simulink model "NDM200_Spindel_Kue_V1"  (Simulink 7.6)
settings: Solver=ode45  StartTime=0.0  StopTime=SimulTime  RelTol=1e-3
values from neighbouring files (symbols this model uses):
  n1 = 380/0.78    (= 487.179487179)    [ParametersGM.m]
  n2 = 1100/0.7    (= 1571.42857143)    [ParametersGM.m]
  p = 500/0.8    (= 625)    [ParametersGM.m]
  sb = 5.67*(10^-8)    (= 5.67e-08)    [ParametersGM.m]
  T_amb = 296    [ParametersGM.m]
  Venti_n2 = 273+40    (= 313)    [ParametersGM.m]
undefined symbols (not defined in the file or in its folder): Job, magnitude, MainDrive, MainDriveCooling
libraries: simulink x1
settings Model: Creator=conid  LastModifiedBy=conid

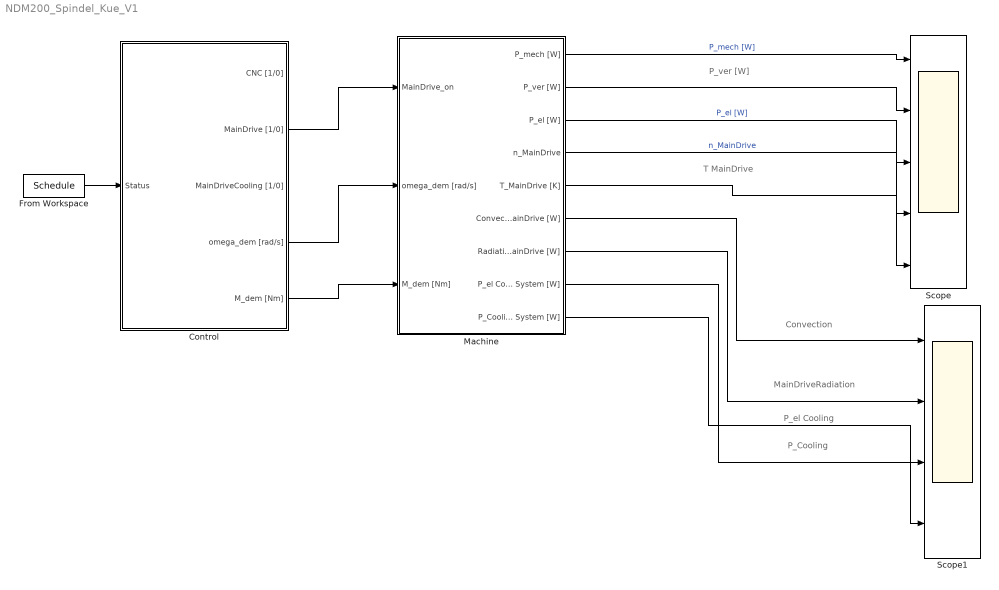
== system NDM200_Spindel_Kue_V1 ==
  note: P_ver [W]
  note: MainDriveRadiation
  note: Convection
  note: T MainDrive
  note: P_el Cooling
  note: P_Cooling
  Control : Subsystem  TreatAsAtomicUnit=on  mask{CNC=[0 1 1 1 1], MainDrive=[0 1 1 1 1], MainDriveCooling=[0 1 1 1 1], Job=Job}
      mask prompts: CNC "Cabinet"; MainDrive "Main Drive"; MainDriveCooling "Main Drive Cooling"; Job "Job Struct"
      mask help:
      | Controls the components of the machine:
      |
      | Status:
      |     0. Off
      |     1. Standby
      |     2. Warmup
      |     3. Setting
      |     4. Machining
      |
      | If the status is machining, the job defined as
      |     - Job.time
      |     - Job.omega_dem
      |     - Job.M_dem
      | will be runned, and repeated.
      mask TabNameString: Status,Status,Status,Job
  From Workspace : FromWorkspace  VariableName=Schedule  SampleTime=0  Interpolate=off  OutputAfterFinalValue=Holding final value
  Machine : Subsystem  TreatAsAtomicUnit=on
  Scope : Scope  NumInputPorts=5
      settings: TickLabels=on  YMin=-5~-5~-5~-5~-5  YMax=5~5~5~5~5  SaveName=Scp_MainDrive
  Scope1 : Scope  NumInputPorts=4
      settings: TickLabels=on  YMin=-5~-5~-5~-5  YMax=5~5~5~5  SaveName=Scp_MainDrive1
  wires:
  Machine/1(P_mech [W]) -> Scope/1  "P_mech [W]"
  Machine/2(P_ver [W]) -> Scope/2
  Machine/3(P_el [W]) -> Scope/3  "P_el [W]"
  Machine/4(n_MainDrive) -> Scope/4  "n_MainDrive"
  From Workspace/1 -> Control/1(Status)
  Control/5(M_dem [Nm]) -> Machine/3(M_dem [Nm])
  Control/4(omega_dem [rad/s]) -> Machine/2(omega_dem [rad/s])
  Control/2(MainDrive [1/0]) -> Machine/1(MainDrive_on)
  Machine/5(T_MainDrive [K]) -> Scope/5
  Machine/6(ConvectionMainDrive [W]) -> Scope1/1
  Machine/7(RadiationMainDrive [W]) -> Scope1/2
  Machine/8(P_el Cooling System [W]) -> Scope1/3
  Machine/9(P_Cooling System [W]) -> Scope1/4

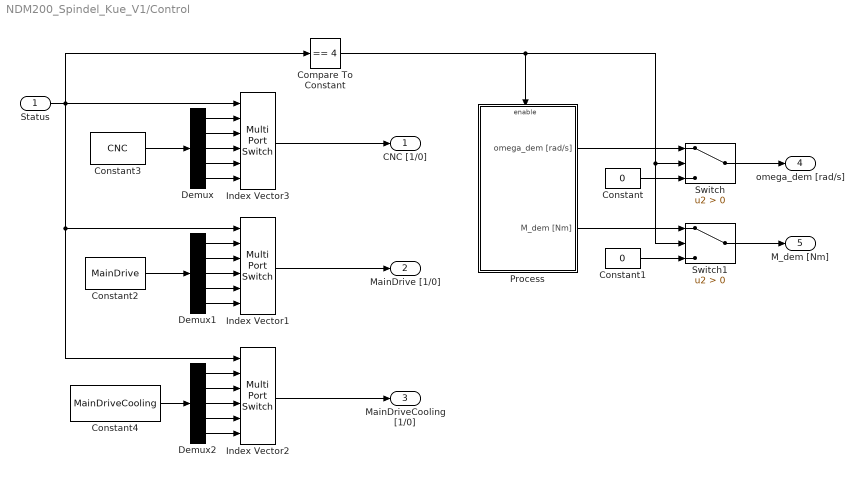
== system NDM200_Spindel_Kue_V1/Control ==
  Status : Inport
  Compare To Constant : simulink/Logic and Bit Operations/Compare To Constant  SystemSampleTime=-1  relop===  const=4  LogicOutDataTypeMode=uint8
  Constant : Constant  Value=0
  Constant1 : Constant  Value=0
  Constant2 : Constant  Value=MainDrive
  Constant3 : Constant  Value=CNC
  Constant4 : Constant  Value=MainDriveCooling
  Demux : Demux  Outputs=5
  Demux1 : Demux  Outputs=5
  Demux2 : Demux  Outputs=5
  Index Vector1 : MultiPortSwitch  DataPortOrder=Zero-based contiguous  Inputs=5  zeroidx=on
  Index Vector2 : MultiPortSwitch  DataPortOrder=Zero-based contiguous  Inputs=5  zeroidx=on
  Index Vector3 : MultiPortSwitch  DataPortOrder=Zero-based contiguous  Inputs=5  zeroidx=on
  Process : Subsystem  TreatAsAtomicUnit=on
  Switch : Switch  Criteria=u2 > Threshold
  Switch1 : Switch  Criteria=u2 > Threshold
  CNC [1/0] : Outport
  MainDrive [1/0] : Outport  Port=2
  MainDriveCooling [1/0] : Outport  Port=3
  omega_dem [rad/s] : Outport  Port=4
  M_dem [Nm] : Outport  Port=5
  wires:
  Status/1 -> Index Vector3/1, Index Vector2/1, Index Vector1/1, Compare To Constant/1
  Demux/1 -> Index Vector3/2
  Demux/2 -> Index Vector3/3
  Demux/3 -> Index Vector3/4
  Demux/4 -> Index Vector3/5
  Demux/5 -> Index Vector3/6
  Index Vector3/1 -> CNC [1/0]/1
  Demux1/1 -> Index Vector1/2
  Demux1/2 -> Index Vector1/3
  Demux1/3 -> Index Vector1/4
  Demux1/4 -> Index Vector1/5
  Demux1/5 -> Index Vector1/6
  Index Vector1/1 -> MainDrive [1/0]/1
  Demux2/1 -> Index Vector2/2
  Demux2/2 -> Index Vector2/3
  Demux2/3 -> Index Vector2/4
  Demux2/4 -> Index Vector2/5
  Demux2/5 -> Index Vector2/6
  Index Vector2/1 -> MainDriveCooling [1/0]/1
  Compare To Constant/1 -> Process/Enable, Switch1/2, Switch/2
  Process/1(omega_dem [rad/s]) -> Switch/1
  Constant/1 -> Switch/3
  Process/2(M_dem [Nm]) -> Switch1/1
  Constant1/1 -> Switch1/3
  Switch/1 -> omega_dem [rad/s]/1
  Switch1/1 -> M_dem [Nm]/1
  Constant3/1 -> Demux/1
  Constant2/1 -> Demux1/1
  Constant4/1 -> Demux2/1

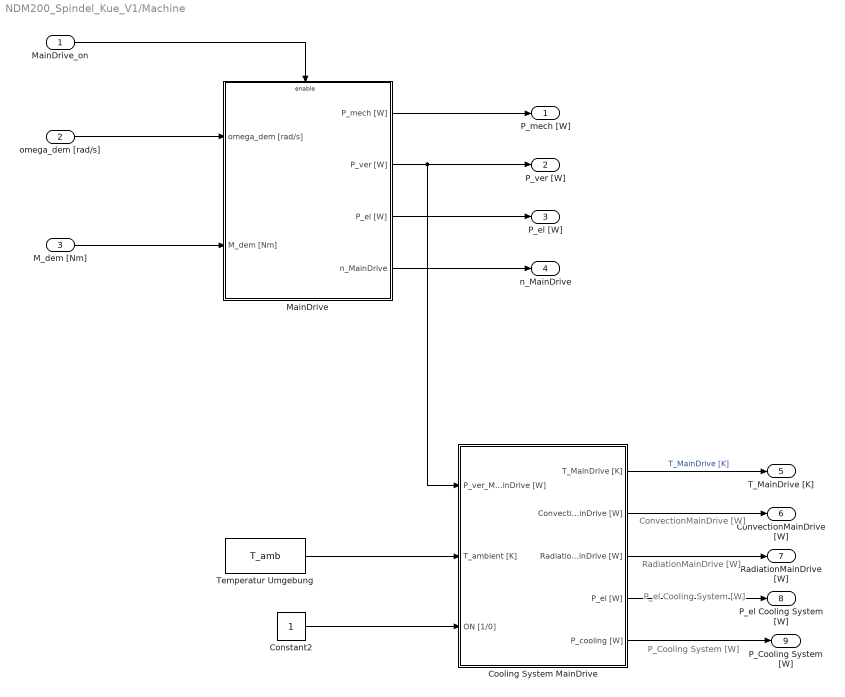
== system NDM200_Spindel_Kue_V1/Machine ==
  note: ConvectionMainDrive [W]
  note: RadiationMainDrive [W]
  note: P_el Cooling System [W]
  note: P_Cooling System [W]
  MainDrive_on : Inport
  omega_dem [rad/s] : Inport  Port=2
  M_dem [Nm] : Inport  Port=3
  Constant2 : Constant
  Cooling System MainDrive : Subsystem  TreatAsAtomicUnit=on
  MainDrive : Subsystem  TreatAsAtomicUnit=on
  Temperatur Umgebung : Constant  Value=T_amb
  P_mech [W] : Outport
  P_ver [W] : Outport  Port=2
  P_el [W] : Outport  Port=3
  n_MainDrive : Outport  Port=4
  T_MainDrive [K] : Outport  Port=5
  ConvectionMainDrive [W] : Outport  Port=6
  RadiationMainDrive [W] : Outport  Port=7
  P_el Cooling System [W] : Outport  Port=8
  P_Cooling System [W] : Outport  Port=9
  wires:
  MainDrive/2(P_ver [W]) -> P_ver [W]/1, Cooling System MainDrive/1(P_ver_MainDrive [W])
  MainDrive/1(P_mech [W]) -> P_mech [W]/1
  MainDrive/3(P_el [W]) -> P_el [W]/1
  MainDrive/4(n_MainDrive) -> n_MainDrive/1
  MainDrive_on/1 -> MainDrive/Enable
  M_dem [Nm]/1 -> MainDrive/2(M_dem [Nm])
  omega_dem [rad/s]/1 -> MainDrive/1(omega_dem [rad/s])
  Temperatur Umgebung/1 -> Cooling System MainDrive/2(T_ambient [K])
  Cooling System MainDrive/1(T_MainDrive [K]) -> T_MainDrive [K]/1  "T_MainDrive [K]"
  Cooling System MainDrive/2(ConvectionMainDrive [W]) -> ConvectionMainDrive [W]/1
  Cooling System MainDrive/3(RadiationMainDrive [W]) -> RadiationMainDrive [W]/1
  Cooling System MainDrive/4(P_el [W]) -> P_el Cooling System [W]/1
  Cooling System MainDrive/5(P_cooling [W]) -> P_Cooling System [W]/1
  Constant2/1 -> Cooling System MainDrive/3(ON [1/0])

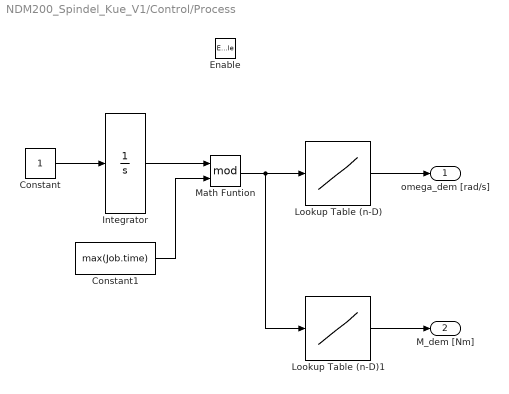
== system NDM200_Spindel_Kue_V1/Control/Process ==
  Enable : EnablePort
  Constant : Constant
  Constant1 : Constant  Value=max(Job.time)
  Integrator : Integrator
  Lookup Table (n-D) : Lookup_n-D  NumberOfTableDimensions=1  BreakpointsForDimension1=Job.time  Table=Job.omega_dem  InterpMethod=None - Flat  ExtrapMethod=Cubic spline  InputSameDT=on
  Lookup Table (n-D)1 : Lookup_n-D  NumberOfTableDimensions=1  BreakpointsForDimension1=Job.time  Table=Job.M_dem  InterpMethod=None - Flat  InputSameDT=on
  Math Funtion : Math  Operator=mod  SaturateOnIntegerOverflow=on
  omega_dem [rad/s] : Outport
  M_dem [Nm] : Outport  Port=2
  wires:
  Constant/1 -> Integrator/1
  Integrator/1 -> Math Funtion/1
  Math Funtion/1 -> Lookup Table (n-D)/1, Lookup Table (n-D)1/1
  Lookup Table (n-D)/1 -> omega_dem [rad/s]/1
  Lookup Table (n-D)1/1 -> M_dem [Nm]/1
  Constant1/1 -> Math Funtion/2

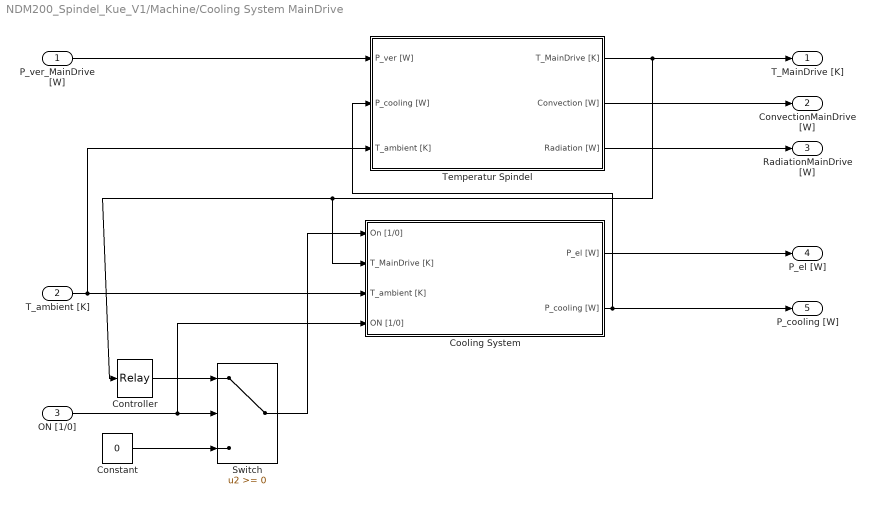
== system NDM200_Spindel_Kue_V1/Machine/Cooling System MainDrive ==
  P_ver_MainDrive [W] : Inport
  T_ambient [K] : Inport  Port=2
  ON [1/0] : Inport  Port=3
  Constant : Constant  Value=0
  Controller : Relay  OnSwitchValue=MainDriveCooling.Tmax  OffSwitchValue=MainDriveCooling.Tmin
  Cooling System : Subsystem
  Switch : Switch
  Temperatur Spindel : Subsystem
  T_MainDrive [K] : Outport
  ConvectionMainDrive [W] : Outport  Port=2
  RadiationMainDrive [W] : Outport  Port=3
  P_el [W] : Outport  Port=4
  P_cooling [W] : Outport  Port=5
  wires:
  P_ver_MainDrive [W]/1 -> Temperatur Spindel/1(P_ver [W])
  Constant/1 -> Switch/3
  ON [1/0]/1 -> Switch/2, Cooling System/4(ON [1/0])
  Controller/1 -> Switch/1
  Temperatur Spindel/1(T_MainDrive [K]) -> Controller/1, Cooling System/2(T_MainDrive [K]), T_MainDrive [K]/1
  Switch/1 -> Cooling System/1(On [1/0])
  T_ambient [K]/1 -> Cooling System/3(T_ambient [K]), Temperatur Spindel/3(T_ambient [K])
  Cooling System/2(P_cooling [W]) -> Temperatur Spindel/2(P_cooling [W]), P_cooling [W]/1
  Temperatur Spindel/2(Convection [W]) -> ConvectionMainDrive [W]/1
  Temperatur Spindel/3(Radiation [W]) -> RadiationMainDrive [W]/1
  Cooling System/1(P_el [W]) -> P_el [W]/1

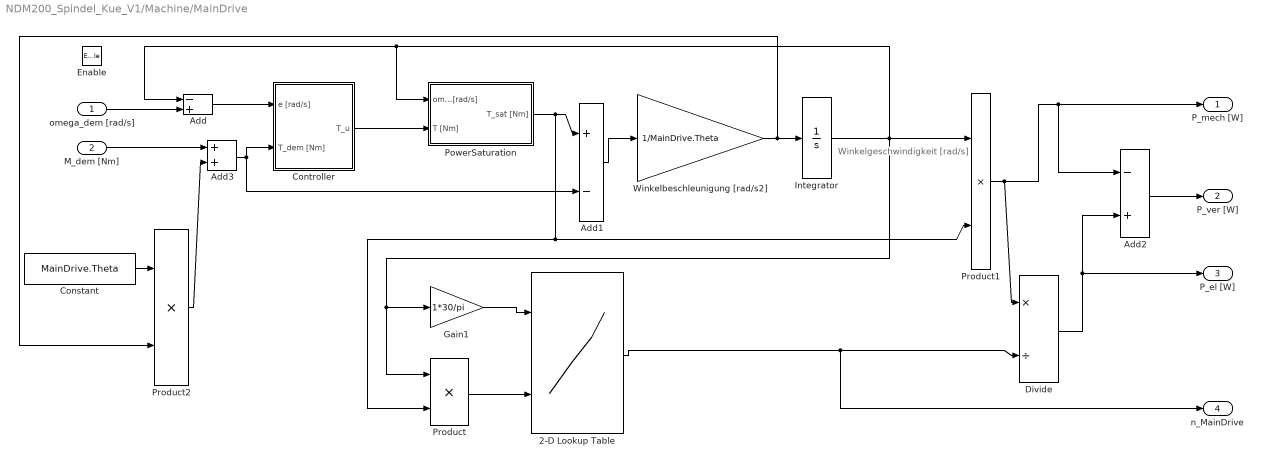
== system NDM200_Spindel_Kue_V1/Machine/MainDrive ==
  note: Winkelgeschwindigkeit [rad/s]
  omega_dem [rad/s] : Inport
  M_dem [Nm] : Inport  Port=2
  Enable : EnablePort
  2-D Lookup Table : Lookup_n-D  BreakpointsForDimension1=MainDrive.Tabelomega  BreakpointsForDimension2=MainDrive.TabelM  Table=MainDrive.Tabeleta  InterpMethod=Cubic spline  ExtrapMethod=Cubic spline  RndMeth=Simplest  InputSameDT=on
  Add : Sum  Inputs=-+
  Add1 : Sum  Inputs=+-
  Add2 : Sum  Inputs=-+
  Add3 : Sum
  Constant : Constant  Value=MainDrive.Theta
  Controller : Subsystem  TreatAsAtomicUnit=on
  Divide : Product  Inputs=*/
  Gain1 : Gain  Gain=1*30/pi
  Integrator : Integrator
  PowerSaturation : Subsystem  TreatAsAtomicUnit=on
  Product : Product  RndMeth=Zero
  Product1 : Product  RndMeth=Zero
  Product2 : Product  RndMeth=Zero
  Winkelbeschleunigung [rad/s2] : Gain  Gain=1/MainDrive.Theta
  P_mech [W] : Outport
  P_ver [W] : Outport  Port=2
  P_el [W] : Outport  Port=3
  n_MainDrive : Outport  Port=4
  wires:
  omega_dem [rad/s]/1 -> Add/2
  Add/1 -> Controller/1(e [rad/s])
  Controller/1(T_u) -> PowerSaturation/2(T [Nm])
  PowerSaturation/1(T_sat [Nm]) -> Add1/1, Product1/2, Product/2
  Add1/1 -> Winkelbeschleunigung [rad/s2]/1
  Winkelbeschleunigung [rad/s2]/1 -> Integrator/1, Product2/2
  Integrator/1 -> Product1/1, Add/1, PowerSaturation/1(omega [rad/s]), Product/1, Gain1/1
  Product1/1 -> Divide/1, P_mech [W]/1, Add2/1
  Add2/1 -> P_ver [W]/1
  Divide/1 -> Add2/2, P_el [W]/1
  2-D Lookup Table/1 -> Divide/2, n_MainDrive/1
  Product/1 -> 2-D Lookup Table/2
  Gain1/1 -> 2-D Lookup Table/1
  Constant/1 -> Product2/1
  Add3/1 -> Controller/2(T_dem [Nm]), Add1/2
  M_dem [Nm]/1 -> Add3/1
  Product2/1 -> Add3/2

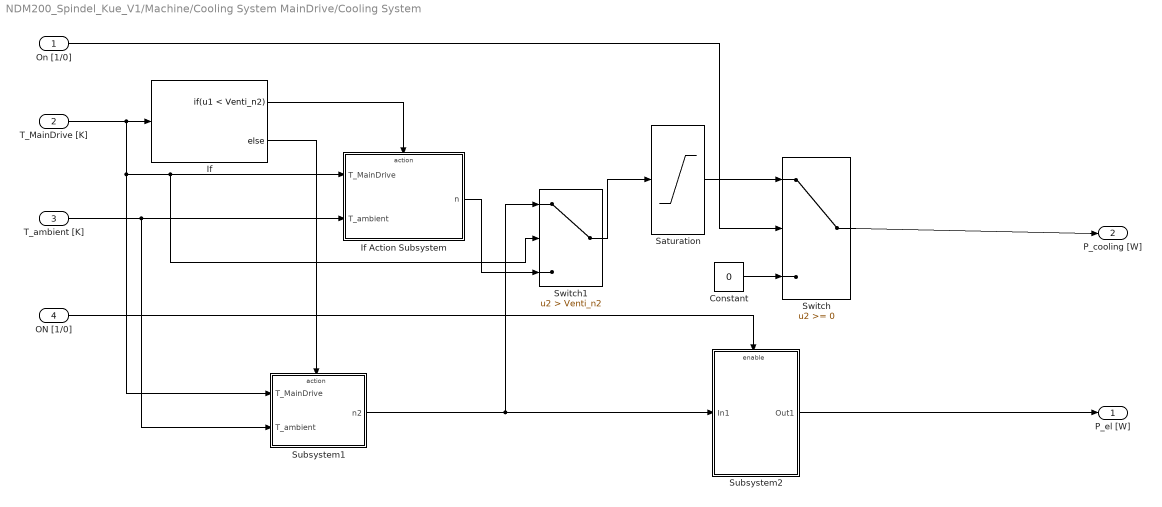
== system NDM200_Spindel_Kue_V1/Machine/Cooling System MainDrive/Cooling System ==
  On [1/0] : Inport
  T_MainDrive [K] : Inport  Port=2
  T_ambient [K] : Inport  Port=3
  ON [1/0] : Inport  Port=4
  Constant : Constant  Value=0
  If : If  IfExpression=u1 < Venti_n2
  If Action Subsystem : Subsystem  TreatAsAtomicUnit=on
  Saturation : Saturate  UpperLimit=12000  LowerLimit=0
  Subsystem1 : Subsystem
  Subsystem2 : Subsystem
  Switch : Switch
  Switch1 : Switch  Criteria=u2 > Threshold  Threshold=Venti_n2
  P_el [W] : Outport
  P_cooling [W] : Outport  Port=2
  wires:
  T_ambient [K]/1 -> Subsystem1/2(T_ambient), If Action Subsystem/2(T_ambient)
  Constant/1 -> Switch/3
  On [1/0]/1 -> Switch/2
  Saturation/1 -> Switch/1
  Switch/1 -> P_cooling [W]/1
  Subsystem2/1(Out1) -> P_el [W]/1
  T_MainDrive [K]/1 -> Subsystem1/1(T_MainDrive), If Action Subsystem/1(T_MainDrive), Switch1/2, If/1
  Subsystem1/1(n2) -> Subsystem2/1(In1), Switch1/1
  ON [1/0]/1 -> Subsystem2/Enable
  Switch1/1 -> Saturation/1
  If/1 -> If Action Subsystem/Action
  If/2 -> Subsystem1/Action
  If Action Subsystem/1(n) -> Switch1/3

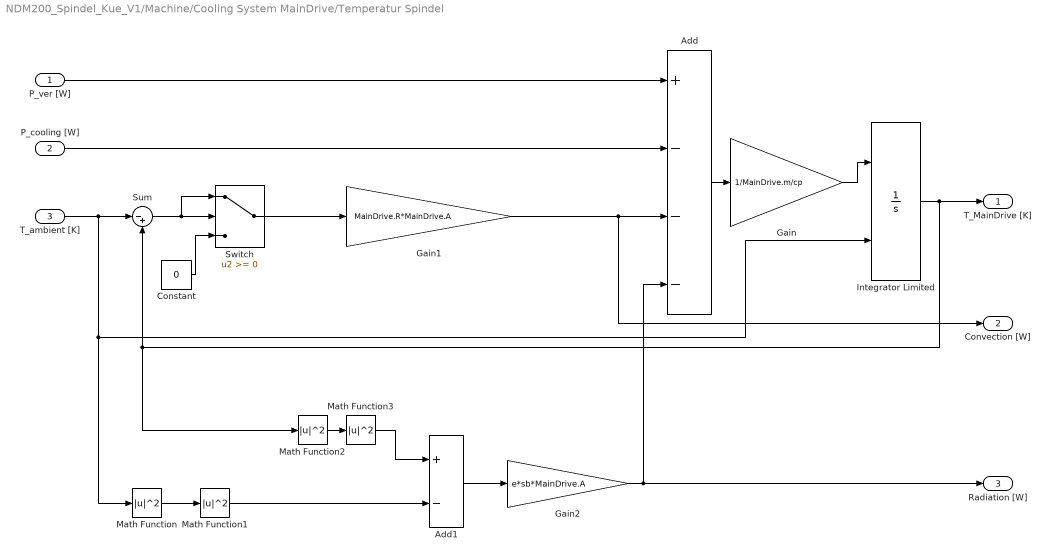
== system NDM200_Spindel_Kue_V1/Machine/Cooling System MainDrive/Temperatur Spindel ==
  P_ver [W] : Inport
  P_cooling [W] : Inport  Port=2
  T_ambient [K] : Inport  Port=3
  Add : Sum  Inputs=+---
  Add1 : Sum  Inputs=+-
  Constant : Constant  Value=0
  Gain : Gain  Gain=1/MainDrive.m/cp
  Gain1 : Gain  Gain=MainDrive.R*MainDrive.A
  Gain2 : Gain  Gain=e*sb*MainDrive.A
  Integrator Limited : Integrator  InitialConditionSource=external  LimitOutput=on
  Math Function{,1..3} (4 alike) : Math  Operator=magnitude^2  SaturateOnIntegerOverflow=on
  Sum : Sum  Inputs=|-+
  Switch : Switch
  T_MainDrive [K] : Outport
  Convection [W] : Outport  Port=2
  Radiation [W] : Outport  Port=3
  wires:
  P_ver [W]/1 -> Add/1
  Gain/1 -> Integrator Limited/1
  Gain1/1 -> Convection [W]/1, Add/3
  Integrator Limited/1 -> T_MainDrive [K]/1, Sum/2, Math Function2/1
  Add/1 -> Gain/1
  Math Function/1 -> Math Function1/1
  Gain2/1 -> Radiation [W]/1, Add/4
  P_cooling [W]/1 -> Add/2
  T_ambient [K]/1 -> Sum/1, Integrator Limited/2, Math Function/1
  Sum/1 -> Switch/2, Switch/1
  Constant/1 -> Switch/3
  Math Function2/1 -> Math Function3/1
  Add1/1 -> Gain2/1
  Math Function3/1 -> Add1/1
  Math Function1/1 -> Add1/2
  Switch/1 -> Gain1/1

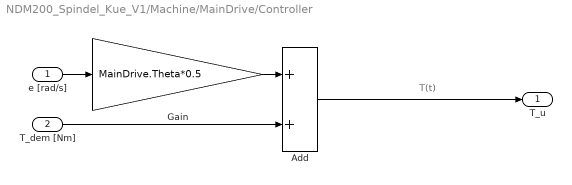
== system NDM200_Spindel_Kue_V1/Machine/MainDrive/Controller ==
  note: T(t)
  e [rad/s] : Inport
  T_dem [Nm] : Inport  Port=2
  Add : Sum
  Gain : Gain  Gain=MainDrive.Theta*0.5
  T_u : Outport
  wires:
  Add/1 -> T_u/1
  T_dem [Nm]/1 -> Add/2
  Gain/1 -> Add/1
  e [rad/s]/1 -> Gain/1

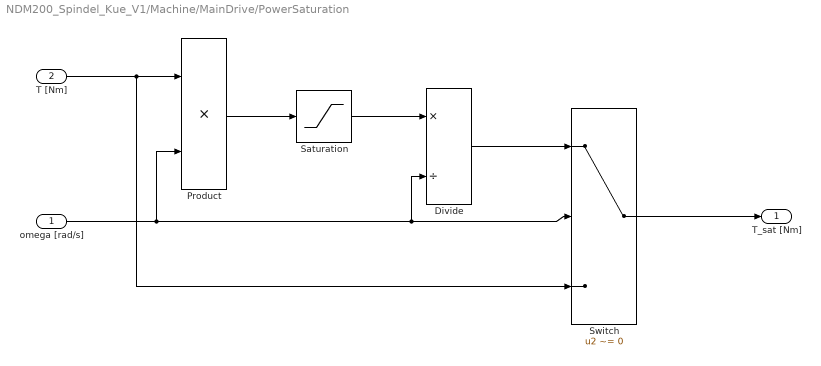
== system NDM200_Spindel_Kue_V1/Machine/MainDrive/PowerSaturation ==
  omega [rad/s] : Inport
  T [Nm] : Inport  Port=2
  Divide : Product  Inputs=*/
  Product : Product  RndMeth=Zero
  Saturation : Saturate  UpperLimit=MainDrive.Pmax  LowerLimit=-MainDrive.Pmax
  Switch : Switch  Criteria=u2 ~= 0
  T_sat [Nm] : Outport
  wires:
  Product/1 -> Saturation/1
  Saturation/1 -> Divide/1
  Divide/1 -> Switch/1
  Switch/1 -> T_sat [Nm]/1
  T [Nm]/1 -> Product/1, Switch/3
  omega [rad/s]/1 -> Switch/2, Divide/2, Product/2

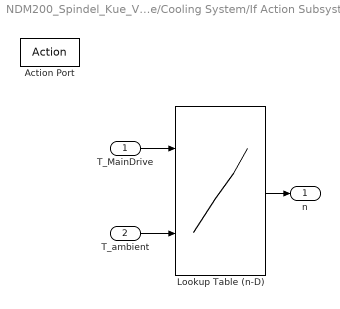
== system NDM200_Spindel_Kue_V1/Machine/Cooling System MainDrive/Cooling System/If Action Subsystem ==
  T_MainDrive : Inport
  T_ambient : Inport  Port=2
  Action Port : ActionPort  ActionType=then
  Lookup Table (n-D) : Lookup_n-D  BreakpointsForDimension1=MainDriveCooling.Air.T_int  BreakpointsForDimension2=MainDriveCooling.Air.T_ext  Table=MainDriveCooling.Air.P  InterpMethod=Cubic spline  ExtrapMethod=None - Clip  InputSameDT=on
  n : Outport
  wires:
  T_ambient/1 -> Lookup Table (n-D)/2
  T_MainDrive/1 -> Lookup Table (n-D)/1
  Lookup Table (n-D)/1 -> n/1

== system NDM200_Spindel_Kue_V1/Machine/Cooling System MainDrive/Cooling System/Subsystem1 ==
  T_MainDrive : Inport
  T_ambient : Inport  Port=2
  Action Port : ActionPort  ActionType=else
  Lookup Table (n-D)1 : Lookup_n-D  BreakpointsForDimension1=MainDriveCooling.Air.T_int  BreakpointsForDimension2=MainDriveCooling.Air.T_ext  Table=MainDriveCooling.Air.P_n2  InterpMethod=Cubic spline  ExtrapMethod=None - Clip  InputSameDT=on
  n2 : Outport
  wires:
  T_ambient/1 -> Lookup Table (n-D)1/2
  T_MainDrive/1 -> Lookup Table (n-D)1/1
  Lookup Table (n-D)1/1 -> n2/1

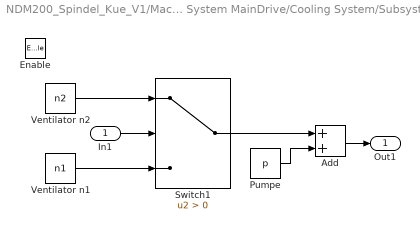
== system NDM200_Spindel_Kue_V1/Machine/Cooling System MainDrive/Cooling System/Subsystem2 ==
  In1 : Inport
  Enable : EnablePort
  Add : Sum
  Pumpe : Constant  Value=p
  Switch1 : Switch  Criteria=u2 > Threshold
  Ventilator n1 : Constant  Value=n1
  Ventilator n2 : Constant  Value=n2
  Out1 : Outport
  wires:
  Switch1/1 -> Add/1
  Ventilator n2/1 -> Switch1/1
  Ventilator n1/1 -> Switch1/3
  Pumpe/1 -> Add/2
  In1/1 -> Switch1/2
  Add/1 -> Out1/1
